simulink model "building_PHPP_v4"  (R2023b)
settings: Solver=ode23tb  StartTime=-building.preruntime+8760*3600  StopTime=building.runtime+8760*3600  EnableMultiTasking=on
PreLoadFcn:
  | tic
StartFcn:
  | pre_time = toc
  | assignin('base','pre_time',pre_time)
  | tic
StopFcn:
  | time = toc
  | assignin('base','time',time)
values from neighbouring files (symbols this model uses):
  A = 7*10*2    (= 140)    [theta_ground_v1.m]    (also in xlswrite1.m = num2cell(data))
  B = A/(0.5 * P)    (= 8.23529411765)    [theta_ground_v1.m]
  building = obj    [BUILDING.m]    (also in create_building_automatic.m = building.save(); ini_building_automatic.m = building.add_variant_hvac(building.variant_hvac, hvac); load_building_automatic.m = building.save())
  C = zeros(1,length(d)+1)    [CONSTRUCTION.m]    (also in DOOR.m = [0 0 0]; WALL.m = [0 0 0]; WINDOW.m = [0 0 0])
  cp = str2num(value)    [CONSTRUCTION.m]
  p = [timevec_weather weather(:,12)]    [BOUNDARY.m]    (also in WEATHER.m = 0; init_carnotUIBK.m = cell2mat(carnotUIBKpaths(i,2)))
  rho = str2num(value)    [CONSTRUCTION.m]    (also in theta_ground_v1.m = 2000)
undefined symbols (not defined in the file or in its folder): Dd, Dreifach, get_building, Qdot_C, Qdot_C_energy, Qdot_H, Qdot_H_energy, Qdot_I_electricity, Qdot_I_electricity_energy, Qdot_I_light, Qdot_I_light_energy, Qdot_I_person, Qdot_I_person_energy, Qdot_S, Qdot_S_energy, Qdot_T_ground, Qdot_T_ground_energy, Qdot_T_neighbour, Qdot_T_neighbour_energy, Qdot_T_opaque, Qdot_T_opaque_energy, Qdot_T_window, Qdot_T_window_energy, Qdot_V_infiltration, Qdot_V_infiltration_energy, Qdot_V_mech, Qdot_V_mech_energy, Qdot_V_window, Qdot_V_window_energy, Tc, Tr, Ts, Wärmeschutzglas, x_CO2, x_H2O, x_VOC
libraries: carnotUIBK x1874, carnot x9, simulink x6
(part 18 of 30)

== system building_PHPP_v4/BUILDING/INTERSECTION_8_9/wall_3 ==
  AIB1 : Inport
  AIB2 : Inport  Port=2
  Qdot_sol1 : Inport  Port=3
  Qdot_sol2 : Inport  Port=4
  EMPTY : carnotUIBK/wall_intersection/EMPTY  VariantControl=(default)
  R-C model : carnotUIBK/wall_intersection/R-C model  VariantControl=V_i_8_9_w3_m1  t0=z.t_ini  d=fliplr(const.parameter.xmesh_beu)  cond=fliplr(const.parameter.lambda)  cwall=fliplr(const.parameter.cp)  rho=fliplr(const.parameter.rho)  reflectground=0.2  abs_emiss=[const.absorption_2 const.emission_2 const.emission_1]  tau=const.parameter.tau  dactive=const.parameter.d_active
      link override alpha_i1/alpha_i_down: VariantControl=V_i_8_9_w3_hti2
      link override alpha_i1/alpha_i_horizontal: VariantControl=V_i_8_9_w3_hti0
      link override alpha_i1/alpha_i_up: VariantControl=V_i_8_9_w3_hti1
      link override alpha_i2/alpha_i_down: VariantControl=V_i_8_9_w3_hti2
      link override alpha_i2/alpha_i_horizontal: VariantControl=V_i_8_9_w3_hti0
      link override alpha_i2/alpha_i_up: VariantControl=V_i_8_9_w3_hti1
  UA : carnotUIBK/wall_intersection/UA  VariantControl=V_i_8_9_w3_m0  U=const.parameter.U
      link override Rsi/down: VariantControl=V_i_8_9_w3_hti2
      link override Rsi/horizontal: VariantControl=V_i_8_9_w3_hti0
      link override Rsi/up: VariantControl=V_i_8_9_w3_hti1
  hygrothermal model : carnotUIBK/wall_intersection/hygrothermal model  VariantControl=V_i_8_9_w3_m2  t0=z.t_ini  reflectground=0.2  abs_emiss=[const.absorption_2 const.emission_2 const.emission_1]  xmesh=const.parameter.xmesh_hygro  X=const.parameter.X  d=const.parameter.d  lambda=const.parameter.lambda_hygro  rho=const.parameter.rho_hygro  cp=const.parameter.cp_hygro  mu=const.parameter.mu  ufs=const.parameter.ufs  FSF_u=const.parameter.FSF_u  FSF_phi=const.parameter.FSF_phi  FSF_dudphi=const.parameter.FSF_dudphi  FSF_k=const.parameter.FSF_k  K_kleff=const.parameter.K_kleff  K_u=const.parameter.K_u  K_kl=const.parameter.K_kl  FSF_length=const.parameter.FSF_length  K_length=const.parameter.K_length  T_ini=const.parameter.T_ini_hygro  Phi_ini=const.parameter.Phi_ini_hygro  T_source=const.parameter.T_source  Phi_source=const.parameter.Phi_source  Tdactive=const.parameter.T_dactive  Phidactive=const.parameter.Phi_dactive
      link override alpha_i1/alpha_i_down: VariantControl=V_i_8_9_w3_hti2
      link override alpha_i1/alpha_i_horizontal: VariantControl=V_i_8_9_w3_hti0
      link override alpha_i1/alpha_i_up: VariantControl=V_i_8_9_w3_hti1
      link override alpha_i2/alpha_i_down: VariantControl=V_i_8_9_w3_hti2
      link override alpha_i2/alpha_i_horizontal: VariantControl=V_i_8_9_w3_hti0
      link override alpha_i2/alpha_i_up: VariantControl=V_i_8_9_w3_hti1
  "[S1]" : Outport  VectorParamsAs1DForOutWhenUnconnected=off
  "[S2]" : Outport  Port=2  VectorParamsAs1DForOutWhenUnconnected=off

== system building_PHPP_v4/BUILDING/INTERSECTION_9_10/airexchange_1 ==
  AIB1 : Inport
  AIB2 : Inport  Port=2
  control : Inport  Port=3
  EMPTY : carnotUIBK/airexchange_intersection/EMPTY  VariantControl=(default)
  airexchange_empiric : carnotUIBK/airexchange_intersection/airexchange_empiric  VariantControl=V_i_9_10_inf1_m0
  airexchange_powerlaw : carnotUIBK/airexchange_intersection/airexchange_powerlaw  VariantControl=V_i_9_10_inf1_m1
  "[S1]" : Outport  VectorParamsAs1DForOutWhenUnconnected=off
  "[S2]" : Outport  Port=2  VectorParamsAs1DForOutWhenUnconnected=off

== system building_PHPP_v4/BUILDING/INTERSECTION_9_10/airexchange_2 ==
  AIB1 : Inport
  AIB2 : Inport  Port=2
  control : Inport  Port=3
  EMPTY : carnotUIBK/airexchange_intersection/EMPTY  VariantControl=(default)
  airexchange_empiric : carnotUIBK/airexchange_intersection/airexchange_empiric  VariantControl=V_i_9_10_inf2_m0
  airexchange_powerlaw : carnotUIBK/airexchange_intersection/airexchange_powerlaw  VariantControl=V_i_9_10_inf2_m1
  "[S1]" : Outport  VectorParamsAs1DForOutWhenUnconnected=off
  "[S2]" : Outport  Port=2  VectorParamsAs1DForOutWhenUnconnected=off

== system building_PHPP_v4/BUILDING/INTERSECTION_9_10/airexchange_3 ==
  AIB1 : Inport
  AIB2 : Inport  Port=2
  control : Inport  Port=3
  EMPTY : carnotUIBK/airexchange_intersection/EMPTY  VariantControl=(default)
  airexchange_empiric : carnotUIBK/airexchange_intersection/airexchange_empiric  VariantControl=V_i_9_10_inf3_m0
  airexchange_powerlaw : carnotUIBK/airexchange_intersection/airexchange_powerlaw  VariantControl=V_i_9_10_inf3_m1
  "[S1]" : Outport  VectorParamsAs1DForOutWhenUnconnected=off
  "[S2]" : Outport  Port=2  VectorParamsAs1DForOutWhenUnconnected=off

== system building_PHPP_v4/BUILDING/INTERSECTION_9_10/wall_1 ==
  AIB1 : Inport
  AIB2 : Inport  Port=2
  Qdot_sol1 : Inport  Port=3
  Qdot_sol2 : Inport  Port=4
  EMPTY : carnotUIBK/wall_intersection/EMPTY  VariantControl=(default)
  R-C model : carnotUIBK/wall_intersection/R-C model  VariantControl=V_i_9_10_w1_m1  t0=z.t_ini  d=fliplr(const.parameter.xmesh_beu)  cond=fliplr(const.parameter.lambda)  cwall=fliplr(const.parameter.cp)  rho=fliplr(const.parameter.rho)  reflectground=0.2  abs_emiss=[const.absorption_2 const.emission_2 const.emission_1]  tau=const.parameter.tau  dactive=const.parameter.d_active
      link override alpha_i1/alpha_i_down: VariantControl=V_i_9_10_w1_hti2
      link override alpha_i1/alpha_i_horizontal: VariantControl=V_i_9_10_w1_hti0
      link override alpha_i1/alpha_i_up: VariantControl=V_i_9_10_w1_hti1
      link override alpha_i2/alpha_i_down: VariantControl=V_i_9_10_w1_hti2
      link override alpha_i2/alpha_i_horizontal: VariantControl=V_i_9_10_w1_hti0
      link override alpha_i2/alpha_i_up: VariantControl=V_i_9_10_w1_hti1
  UA : carnotUIBK/wall_intersection/UA  VariantControl=V_i_9_10_w1_m0  U=const.parameter.U
      link override Rsi/down: VariantControl=V_i_9_10_w1_hti2
      link override Rsi/horizontal: VariantControl=V_i_9_10_w1_hti0
      link override Rsi/up: VariantControl=V_i_9_10_w1_hti1
  hygrothermal model : carnotUIBK/wall_intersection/hygrothermal model  VariantControl=V_i_9_10_w1_m2  t0=z.t_ini  reflectground=0.2  abs_emiss=[const.absorption_2 const.emission_2 const.emission_1]  xmesh=const.parameter.xmesh_hygro  X=const.parameter.X  d=const.parameter.d  lambda=const.parameter.lambda_hygro  rho=const.parameter.rho_hygro  cp=const.parameter.cp_hygro  mu=const.parameter.mu  ufs=const.parameter.ufs  FSF_u=const.parameter.FSF_u  FSF_phi=const.parameter.FSF_phi  FSF_dudphi=const.parameter.FSF_dudphi  FSF_k=const.parameter.FSF_k  K_kleff=const.parameter.K_kleff  K_u=const.parameter.K_u  K_kl=const.parameter.K_kl  FSF_length=const.parameter.FSF_length  K_length=const.parameter.K_length  T_ini=const.parameter.T_ini_hygro  Phi_ini=const.parameter.Phi_ini_hygro  T_source=const.parameter.T_source  Phi_source=const.parameter.Phi_source  Tdactive=const.parameter.T_dactive  Phidactive=const.parameter.Phi_dactive
      link override alpha_i1/alpha_i_down: VariantControl=V_i_9_10_w1_hti2
      link override alpha_i1/alpha_i_horizontal: VariantControl=V_i_9_10_w1_hti0
      link override alpha_i1/alpha_i_up: VariantControl=V_i_9_10_w1_hti1
      link override alpha_i2/alpha_i_down: VariantControl=V_i_9_10_w1_hti2
      link override alpha_i2/alpha_i_horizontal: VariantControl=V_i_9_10_w1_hti0
      link override alpha_i2/alpha_i_up: VariantControl=V_i_9_10_w1_hti1
  "[S1]" : Outport  VectorParamsAs1DForOutWhenUnconnected=off
  "[S2]" : Outport  Port=2  VectorParamsAs1DForOutWhenUnconnected=off

== system building_PHPP_v4/BUILDING/INTERSECTION_9_10/wall_2 ==
  AIB1 : Inport
  AIB2 : Inport  Port=2
  Qdot_sol1 : Inport  Port=3
  Qdot_sol2 : Inport  Port=4
  EMPTY : carnotUIBK/wall_intersection/EMPTY  VariantControl=(default)
  R-C model : carnotUIBK/wall_intersection/R-C model  VariantControl=V_i_9_10_w2_m1  t0=z.t_ini  d=fliplr(const.parameter.xmesh_beu)  cond=fliplr(const.parameter.lambda)  cwall=fliplr(const.parameter.cp)  rho=fliplr(const.parameter.rho)  reflectground=0.2  abs_emiss=[const.absorption_2 const.emission_2 const.emission_1]  tau=const.parameter.tau  dactive=const.parameter.d_active
      link override alpha_i1/alpha_i_down: VariantControl=V_i_9_10_w2_hti2
      link override alpha_i1/alpha_i_horizontal: VariantControl=V_i_9_10_w2_hti0
      link override alpha_i1/alpha_i_up: VariantControl=V_i_9_10_w2_hti1
      link override alpha_i2/alpha_i_down: VariantControl=V_i_9_10_w2_hti2
      link override alpha_i2/alpha_i_horizontal: VariantControl=V_i_9_10_w2_hti0
      link override alpha_i2/alpha_i_up: VariantControl=V_i_9_10_w2_hti1
  UA : carnotUIBK/wall_intersection/UA  VariantControl=V_i_9_10_w2_m0  U=const.parameter.U
      link override Rsi/down: VariantControl=V_i_9_10_w2_hti2
      link override Rsi/horizontal: VariantControl=V_i_9_10_w2_hti0
      link override Rsi/up: VariantControl=V_i_9_10_w2_hti1
  hygrothermal model : carnotUIBK/wall_intersection/hygrothermal model  VariantControl=V_i_9_10_w2_m2  t0=z.t_ini  reflectground=0.2  abs_emiss=[const.absorption_2 const.emission_2 const.emission_1]  xmesh=const.parameter.xmesh_hygro  X=const.parameter.X  d=const.parameter.d  lambda=const.parameter.lambda_hygro  rho=const.parameter.rho_hygro  cp=const.parameter.cp_hygro  mu=const.parameter.mu  ufs=const.parameter.ufs  FSF_u=const.parameter.FSF_u  FSF_phi=const.parameter.FSF_phi  FSF_dudphi=const.parameter.FSF_dudphi  FSF_k=const.parameter.FSF_k  K_kleff=const.parameter.K_kleff  K_u=const.parameter.K_u  K_kl=const.parameter.K_kl  FSF_length=const.parameter.FSF_length  K_length=const.parameter.K_length  T_ini=const.parameter.T_ini_hygro  Phi_ini=const.parameter.Phi_ini_hygro  T_source=const.parameter.T_source  Phi_source=const.parameter.Phi_source  Tdactive=const.parameter.T_dactive  Phidactive=const.parameter.Phi_dactive
      link override alpha_i1/alpha_i_down: VariantControl=V_i_9_10_w2_hti2
      link override alpha_i1/alpha_i_horizontal: VariantControl=V_i_9_10_w2_hti0
      link override alpha_i1/alpha_i_up: VariantControl=V_i_9_10_w2_hti1
      link override alpha_i2/alpha_i_down: VariantControl=V_i_9_10_w2_hti2
      link override alpha_i2/alpha_i_horizontal: VariantControl=V_i_9_10_w2_hti0
      link override alpha_i2/alpha_i_up: VariantControl=V_i_9_10_w2_hti1
  "[S1]" : Outport  VectorParamsAs1DForOutWhenUnconnected=off
  "[S2]" : Outport  Port=2  VectorParamsAs1DForOutWhenUnconnected=off

== system building_PHPP_v4/BUILDING/INTERSECTION_9_10/wall_3 ==
  AIB1 : Inport
  AIB2 : Inport  Port=2
  Qdot_sol1 : Inport  Port=3
  Qdot_sol2 : Inport  Port=4
  EMPTY : carnotUIBK/wall_intersection/EMPTY  VariantControl=(default)
  R-C model : carnotUIBK/wall_intersection/R-C model  VariantControl=V_i_9_10_w3_m1  t0=z.t_ini  d=fliplr(const.parameter.xmesh_beu)  cond=fliplr(const.parameter.lambda)  cwall=fliplr(const.parameter.cp)  rho=fliplr(const.parameter.rho)  reflectground=0.2  abs_emiss=[const.absorption_2 const.emission_2 const.emission_1]  tau=const.parameter.tau  dactive=const.parameter.d_active
      link override alpha_i1/alpha_i_down: VariantControl=V_i_9_10_w3_hti2
      link override alpha_i1/alpha_i_horizontal: VariantControl=V_i_9_10_w3_hti0
      link override alpha_i1/alpha_i_up: VariantControl=V_i_9_10_w3_hti1
      link override alpha_i2/alpha_i_down: VariantControl=V_i_9_10_w3_hti2
      link override alpha_i2/alpha_i_horizontal: VariantControl=V_i_9_10_w3_hti0
      link override alpha_i2/alpha_i_up: VariantControl=V_i_9_10_w3_hti1
  UA : carnotUIBK/wall_intersection/UA  VariantControl=V_i_9_10_w3_m0  U=const.parameter.U
      link override Rsi/down: VariantControl=V_i_9_10_w3_hti2
      link override Rsi/horizontal: VariantControl=V_i_9_10_w3_hti0
      link override Rsi/up: VariantControl=V_i_9_10_w3_hti1
  hygrothermal model : carnotUIBK/wall_intersection/hygrothermal model  VariantControl=V_i_9_10_w3_m2  t0=z.t_ini  reflectground=0.2  abs_emiss=[const.absorption_2 const.emission_2 const.emission_1]  xmesh=const.parameter.xmesh_hygro  X=const.parameter.X  d=const.parameter.d  lambda=const.parameter.lambda_hygro  rho=const.parameter.rho_hygro  cp=const.parameter.cp_hygro  mu=const.parameter.mu  ufs=const.parameter.ufs  FSF_u=const.parameter.FSF_u  FSF_phi=const.parameter.FSF_phi  FSF_dudphi=const.parameter.FSF_dudphi  FSF_k=const.parameter.FSF_k  K_kleff=const.parameter.K_kleff  K_u=const.parameter.K_u  K_kl=const.parameter.K_kl  FSF_length=const.parameter.FSF_length  K_length=const.parameter.K_length  T_ini=const.parameter.T_ini_hygro  Phi_ini=const.parameter.Phi_ini_hygro  T_source=const.parameter.T_source  Phi_source=const.parameter.Phi_source  Tdactive=const.parameter.T_dactive  Phidactive=const.parameter.Phi_dactive
      link override alpha_i1/alpha_i_down: VariantControl=V_i_9_10_w3_hti2
      link override alpha_i1/alpha_i_horizontal: VariantControl=V_i_9_10_w3_hti0
      link override alpha_i1/alpha_i_up: VariantControl=V_i_9_10_w3_hti1
      link override alpha_i2/alpha_i_down: VariantControl=V_i_9_10_w3_hti2
      link override alpha_i2/alpha_i_horizontal: VariantControl=V_i_9_10_w3_hti0
      link override alpha_i2/alpha_i_up: VariantControl=V_i_9_10_w3_hti1
  "[S1]" : Outport  VectorParamsAs1DForOutWhenUnconnected=off
  "[S2]" : Outport  Port=2  VectorParamsAs1DForOutWhenUnconnected=off

== system building_PHPP_v4/BUILDING/ZONE_1/gain_1 ==
  AIB : Inport
  control : Inport  Port=2
  EMPTY : carnotUIBK/gain/EMPTY  SystemSampleTime=-1  VariantControl=(default)
  Equipment : carnotUIBK/gain/Equipment  SystemSampleTime=-1  VariantControl=V_z1_i1_m2
  Light : carnotUIBK/gain/Light  SystemSampleTime=-1  VariantControl=V_z1_i1_m1
  Moisture : carnotUIBK/gain/Moisture  SystemSampleTime=-1  VariantControl=V_z1_i1_m3
  People : carnotUIBK/gain/People  SystemSampleTime=-1  VariantControl=V_z1_i1_m0  VariantActivationTime=update diagram  AllowFlexibleInterface=on  Latency=0  AutoFrameSizeCalculation=off
  "[S]" : Outport  VectorParamsAs1DForOutWhenUnconnected=off

== system building_PHPP_v4/BUILDING/ZONE_1/gain_2 ==
  AIB : Inport
  control : Inport  Port=2
  EMPTY : carnotUIBK/gain/EMPTY  SystemSampleTime=-1  VariantControl=(default)  VariantActivationTime=update diagram  AllowFlexibleInterface=on  Latency=0  AutoFrameSizeCalculation=off
  Equipment : carnotUIBK/gain/Equipment  SystemSampleTime=-1  VariantControl=V_z1_i2_m2
  Light : carnotUIBK/gain/Light  SystemSampleTime=-1  VariantControl=V_z1_i2_m1
  Moisture : carnotUIBK/gain/Moisture  SystemSampleTime=-1  VariantControl=V_z1_i2_m3
  People : carnotUIBK/gain/People  SystemSampleTime=-1  VariantControl=V_z1_i2_m0
  "[S]" : Outport  VectorParamsAs1DForOutWhenUnconnected=off

== system building_PHPP_v4/BUILDING/ZONE_1/gain_3 ==
  AIB : Inport
  control : Inport  Port=2
  EMPTY : carnotUIBK/gain/EMPTY  SystemSampleTime=-1  VariantControl=(default)  VariantActivationTime=update diagram  AllowFlexibleInterface=on  Latency=0  AutoFrameSizeCalculation=off
  Equipment : carnotUIBK/gain/Equipment  SystemSampleTime=-1  VariantControl=V_z1_i3_m2
  Light : carnotUIBK/gain/Light  SystemSampleTime=-1  VariantControl=V_z1_i3_m1
  Moisture : carnotUIBK/gain/Moisture  SystemSampleTime=-1  VariantControl=V_z1_i3_m3
  People : carnotUIBK/gain/People  SystemSampleTime=-1  VariantControl=V_z1_i3_m0
  "[S]" : Outport  VectorParamsAs1DForOutWhenUnconnected=off

== system building_PHPP_v4/BUILDING/ZONE_1/gain_4 ==
  AIB : Inport
  control : Inport  Port=2
  EMPTY : carnotUIBK/gain/EMPTY  SystemSampleTime=-1  VariantControl=(default)  VariantActivationTime=update diagram  AllowFlexibleInterface=on  Latency=0  AutoFrameSizeCalculation=off
  Equipment : carnotUIBK/gain/Equipment  SystemSampleTime=-1  VariantControl=V_z1_i4_m2
  Light : carnotUIBK/gain/Light  SystemSampleTime=-1  VariantControl=V_z1_i4_m1
  Moisture : carnotUIBK/gain/Moisture  SystemSampleTime=-1  VariantControl=V_z1_i4_m3
  People : carnotUIBK/gain/People  SystemSampleTime=-1  VariantControl=V_z1_i4_m0
  "[S]" : Outport  VectorParamsAs1DForOutWhenUnconnected=off

== system building_PHPP_v4/BUILDING/ZONE_1/gain_5 ==
  AIB : Inport
  control : Inport  Port=2
  EMPTY : carnotUIBK/gain/EMPTY  SystemSampleTime=-1  VariantControl=(default)  VariantActivationTime=update diagram  AllowFlexibleInterface=on  Latency=0  AutoFrameSizeCalculation=off
  Equipment : carnotUIBK/gain/Equipment  SystemSampleTime=-1  VariantControl=V_z1_i5_m2
  Light : carnotUIBK/gain/Light  SystemSampleTime=-1  VariantControl=V_z1_i5_m1
  Moisture : carnotUIBK/gain/Moisture  SystemSampleTime=-1  VariantControl=V_z1_i5_m3
  People : carnotUIBK/gain/People  SystemSampleTime=-1  VariantControl=V_z1_i5_m0
  "[S]" : Outport  VectorParamsAs1DForOutWhenUnconnected=off

== system building_PHPP_v4/BUILDING/ZONE_1/infiltration_1 ==
  AIB : Inport
  WDB : Inport  Port=2
  control : Inport  Port=3
  EMPTY : carnotUIBK/infiltration/EMPTY  VariantControl=(default)
  infiltration_constant : carnotUIBK/infiltration/infiltration_constant  VariantControl=V_z1_inf1_m0  volume=z.heated_volume  n50=z.n50  wind_e=0.07  co2=400
  infiltration_pressure : carnotUIBK/infiltration/infiltration_pressure  VariantControl=V_z1_inf1_m1  volume=z.heated_volume  n50=z.n50  wind_e=0.07  co2=400
  "[S]" : Outport  VectorParamsAs1DForOutWhenUnconnected=off

== system building_PHPP_v4/BUILDING/ZONE_1/infiltration_2 ==
  AIB : Inport
  WDB : Inport  Port=2
  control : Inport  Port=3
  EMPTY : carnotUIBK/infiltration/EMPTY  VariantControl=(default)
  infiltration_constant : carnotUIBK/infiltration/infiltration_constant  VariantControl=V_z1_inf2_m0  volume=z.heated_volume  n50=z.n50  wind_e=0.07  co2=400
  infiltration_pressure : carnotUIBK/infiltration/infiltration_pressure  VariantControl=V_z1_inf2_m1  volume=z.heated_volume  n50=z.n50  wind_e=0.07  co2=400
  "[S]" : Outport  VectorParamsAs1DForOutWhenUnconnected=off

== system building_PHPP_v4/BUILDING/ZONE_1/infiltration_3 ==
  AIB : Inport
  WDB : Inport  Port=2
  control : Inport  Port=3
  EMPTY : carnotUIBK/infiltration/EMPTY  VariantControl=(default)
  infiltration_constant : carnotUIBK/infiltration/infiltration_constant  VariantControl=V_z1_inf3_m0  volume=z.heated_volume  n50=z.n50  wind_e=0.07  co2=400
  infiltration_pressure : carnotUIBK/infiltration/infiltration_pressure  VariantControl=V_z1_inf3_m1  volume=z.heated_volume  n50=z.n50  wind_e=0.07  co2=400
  "[S]" : Outport  VectorParamsAs1DForOutWhenUnconnected=off

== system building_PHPP_v4/BUILDING/ZONE_1/infiltration_4 ==
  AIB : Inport
  WDB : Inport  Port=2
  control : Inport  Port=3
  EMPTY : carnotUIBK/infiltration/EMPTY  VariantControl=(default)
  infiltration_constant : carnotUIBK/infiltration/infiltration_constant  VariantControl=V_z1_inf4_m0  volume=z.heated_volume  n50=z.n50  wind_e=0.07  co2=400
  infiltration_pressure : carnotUIBK/infiltration/infiltration_pressure  VariantControl=V_z1_inf4_m1  volume=z.heated_volume  n50=z.n50  wind_e=0.07  co2=400
  "[S]" : Outport  VectorParamsAs1DForOutWhenUnconnected=off

== system building_PHPP_v4/BUILDING/ZONE_1/infiltration_5 ==
  AIB : Inport
  WDB : Inport  Port=2
  control : Inport  Port=3
  EMPTY : carnotUIBK/infiltration/EMPTY  VariantControl=(default)
  infiltration_constant : carnotUIBK/infiltration/infiltration_constant  VariantControl=V_z1_inf5_m0  volume=z.heated_volume  n50=z.n50  wind_e=0.07  co2=400
  infiltration_pressure : carnotUIBK/infiltration/infiltration_pressure  VariantControl=V_z1_inf5_m1  volume=z.heated_volume  n50=z.n50  wind_e=0.07  co2=400
  "[S]" : Outport  VectorParamsAs1DForOutWhenUnconnected=off

== system building_PHPP_v4/BUILDING/ZONE_1/room_node ==
  sum([S]) : Inport
  1-node : carnotUIBK/room_node/1-node  VariantControl=V_z1_m2  zoneairvolume=z.heated_volume  zoneheight=z.heated_volume/z.heated_area  zonestartTEMP=z.t_ini  zonestartWATER=z.phi_ini  zonestartCO2=z.CO2_ini  zonestartVOC=z.VOC_ini  zonestartP0=1e5/(293.15)*(273.15+z.t_ini)  timeconst=z.timeconstant  mcp=z.cp_spec*z.heated_area
  1-node_womass : carnotUIBK/room_node/1-node_womass  VariantControl=V_z1_m4  zoneairvolume=z.heated_volume  zoneheight=z.heated_volume/z.heated_area  zonestartTEMP=z.t_ini  zonestartWATER=z.phi_ini  zonestartCO2=z.CO2_ini  zonestartVOC=z.VOC_ini  zonestartP0=1e5/(293.15)*(273.15+z.t_ini)  timeconst=z.timeconstant  mcp=z.cp_spec*z.heated_area
  2-node : carnotUIBK/room_node/2-node  VariantControl=V_z1_m3  zoneairvolume=z.heated_volume  zoneheight=z.heated_volume/z.heated_area  zonestartTEMP=z.t_ini  zonestartWATER=z.phi_ini  zonestartCO2=z.CO2_ini  zonestartVOC=z.VOC_ini  zonestartP0=1e5/(293.15)*(273.15+z.t_ini)  timeconst=z.timeconstant
  2-node_ideal : carnotUIBK/room_node/2-node_ideal  VariantControl=V_z1_m1  zoneairvolume=z.heated_volume  zoneheight=z.heated_volume/z.heated_area  zonestartTEMP=z.t_ini  zonestartWATER=z.phi_ini  zonestartCO2=z.CO2_ini  zonestartVOC=z.VOC_ini  zonestartP0=1e5/(293.15)*(273.15+z.t_ini)  timeconst=z.timeconstant  temperature_timevalues=z.profile_timevalues  temperature_timeduration=z.profile_timeduration  temperature_Tc=z.profile_Tc  temperature_Tr=z.profile_Tc
  EMPTY : carnotUIBK/room_node/EMPTY  VariantControl=(default)  temperature_timevalues=z.profile_timevalues  temperature_timeduration=z.profile_timeduration  temperature_Tc=z.profile_Tc  temperature_Tr=z.profile_Tr  temperature_rH=z.profile_rH  temperature_CO2=z.profile_CO2  temperature_VOC=z.profile_VOC  temperature_p=z.profile_p
  BDB : Outport  VectorParamsAs1DForOutWhenUnconnected=off
  AIB : Outport  Port=2  VectorParamsAs1DForOutWhenUnconnected=off
  Qdot_sol : Outport  Port=3  VectorParamsAs1DForOutWhenUnconnected=off

== system building_PHPP_v4/BUILDING/ZONE_1/wall_1 ==
  WDB : Inport
  GDB : Inport  Port=2
  NDB : Inport  Port=3
  AIB : Inport  Port=4
  Qdot_in : Inport  Port=5
  Qdot_sol : Inport  Port=6
  EMPTY : carnotUIBK/wall_zone/EMPTY  VariantControl=(default)
  R-C model : carnotUIBK/wall_zone/R-C model  VariantControl=V_z1_w1_m1  t0=z.t_ini  d=fliplr(const.parameter.xmesh_beu)  cond=fliplr(const.parameter.lambda)  cwall=fliplr(const.parameter.cp)  rho=fliplr(const.parameter.rho)  reflectground=0.2  abs_emiss=[const.absorption_2 const.emission_2 const.emission_1]  tau=const.parameter.tau  dactive=const.parameter.d_active
      link override alpha_e/alpha_e_AMBIENT: VariantControl=V_z1_w1_hte0
      link override alpha_e/alpha_e_GROUND: VariantControl=V_z1_w1_hte1
      link override alpha_e/alpha_e_INTERNAL: VariantControl=V_z1_w1_hte2
      link override alpha_e/alpha_e_INTERNAL/alpha_i/alpha_i_down: VariantControl=V_z1_w1_hti2
      link override alpha_e/alpha_e_INTERNAL/alpha_i/alpha_i_horizontal: VariantControl=V_z1_w1_hti0
      link override alpha_e/alpha_e_INTERNAL/alpha_i/alpha_i_up: VariantControl=V_z1_w1_hti1
      link override alpha_e/alpha_e_NEIGHBOUR: VariantControl=V_z1_w1_hte3
      link override alpha_e/alpha_e_NEIGHBOUR/alpha_i/alpha_i_down: VariantControl=V_z1_w1_hti2
      link override alpha_e/alpha_e_NEIGHBOUR/alpha_i/alpha_i_horizontal: VariantControl=V_z1_w1_hti0
      link override alpha_e/alpha_e_NEIGHBOUR/alpha_i/alpha_i_up: VariantControl=V_z1_w1_hti1
      link override alpha_i/alpha_i_down: VariantControl=V_z1_w1_hti2
      link override alpha_i/alpha_i_horizontal: VariantControl=V_z1_w1_hti0
      link override alpha_i/alpha_i_up: VariantControl=V_z1_w1_hti1
  UA : carnotUIBK/wall_zone/UA  VariantControl=V_z1_w1_m0  U=const.parameter.U
      link override Rse/AMBIENT: VariantControl=V_z1_w1_hte0
      link override Rse/GROUND: VariantControl=V_z1_w1_hte1
      link override Rse/INTERNAL: VariantControl=V_z1_w1_hte2
      link override Rse/NEIGHBOUR: VariantControl=V_z1_w1_hte3
      link override Rsi/down: VariantControl=V_z1_w1_hti2
      link override Rsi/horizontal: VariantControl=V_z1_w1_hti0
      link override Rsi/up: VariantControl=V_z1_w1_hti1
  hygrothermal model : carnotUIBK/wall_zone/hygrothermal model  VariantControl=V_z1_w1_m2  t0=z.t_ini  reflectground=0.2  abs_emiss=[const.absorption_2 const.emission_2 const.emission_1]  xmesh=const.parameter.xmesh_hygro  X=const.parameter.X  d=const.parameter.d  lambda=const.parameter.lambda_hygro  rho=const.parameter.rho_hygro  cp=const.parameter.cp_hygro  mu=const.parameter.mu  ufs=const.parameter.ufs  FSF_u=const.parameter.FSF_u  FSF_phi=const.parameter.FSF_phi  FSF_dudphi=const.parameter.FSF_dudphi  FSF_k=const.parameter.FSF_k  K_kleff=const.parameter.K_kleff  K_u=const.parameter.K_u  K_kl=const.parameter.K_kl  FSF_length=const.parameter.FSF_length  K_length=const.parameter.K_length  T_ini=const.parameter.T_ini_hygro  Phi_ini=const.parameter.Phi_ini_hygro  T_source=const.parameter.T_source  Phi_source=const.parameter.Phi_source  Tdactive=const.parameter.T_dactive  Phidactive=const.parameter.Phi_dactive
      link override alpha_e/alpha_e_AMBIENT: VariantControl=V_z1_w1_hte0
      link override alpha_e/alpha_e_GROUND: VariantControl=V_z1_w1_hte1
      link override alpha_e/alpha_e_INTERNAL: VariantControl=V_z1_w1_hte2
      link override alpha_e/alpha_e_INTERNAL/alpha_i/alpha_i_down: VariantControl=V_z1_w1_hti2
      link override alpha_e/alpha_e_INTERNAL/alpha_i/alpha_i_horizontal: VariantControl=V_z1_w1_hti0
      link override alpha_e/alpha_e_INTERNAL/alpha_i/alpha_i_up: VariantControl=V_z1_w1_hti1
      link override alpha_e/alpha_e_NEIGHBOUR: VariantControl=V_z1_w1_hte3
      link override alpha_e/alpha_e_NEIGHBOUR/alpha_i/alpha_i_down: VariantControl=V_z1_w1_hti2
      link override alpha_e/alpha_e_NEIGHBOUR/alpha_i/alpha_i_horizontal: VariantControl=V_z1_w1_hti0
      link override alpha_e/alpha_e_NEIGHBOUR/alpha_i/alpha_i_up: VariantControl=V_z1_w1_hti1
      link override alpha_i/alpha_i_down: VariantControl=V_z1_w1_hti2
      link override alpha_i/alpha_i_horizontal: VariantControl=V_z1_w1_hti0
      link override alpha_i/alpha_i_up: VariantControl=V_z1_w1_hti1
  "[S]" : Outport  VectorParamsAs1DForOutWhenUnconnected=off
  theta_out : Outport  Port=2  VectorParamsAs1DForOutWhenUnconnected=off

== system building_PHPP_v4/BUILDING/ZONE_1/wall_10 ==
  WDB : Inport
  GDB : Inport  Port=2
  NDB : Inport  Port=3
  AIB : Inport  Port=4
  Qdot_in : Inport  Port=5
  Qdot_sol : Inport  Port=6
  EMPTY : carnotUIBK/wall_zone/EMPTY  VariantControl=(default)
  R-C model : carnotUIBK/wall_zone/R-C model  VariantControl=V_z1_w10_m1  t0=z.t_ini  d=fliplr(const.parameter.xmesh_beu)  cond=fliplr(const.parameter.lambda)  cwall=fliplr(const.parameter.cp)  rho=fliplr(const.parameter.rho)  reflectground=0.2  abs_emiss=[const.absorption_2 const.emission_2 const.emission_1]  tau=const.parameter.tau  dactive=const.parameter.d_active
      link override alpha_e/alpha_e_AMBIENT: VariantControl=V_z1_w10_hte0
      link override alpha_e/alpha_e_GROUND: VariantControl=V_z1_w10_hte1
      link override alpha_e/alpha_e_INTERNAL: VariantControl=V_z1_w10_hte2
      link override alpha_e/alpha_e_INTERNAL/alpha_i/alpha_i_down: VariantControl=V_z1_w10_hti2
      link override alpha_e/alpha_e_INTERNAL/alpha_i/alpha_i_horizontal: VariantControl=V_z1_w10_hti0
      link override alpha_e/alpha_e_INTERNAL/alpha_i/alpha_i_up: VariantControl=V_z1_w10_hti1
      link override alpha_e/alpha_e_NEIGHBOUR: VariantControl=V_z1_w10_hte3
      link override alpha_e/alpha_e_NEIGHBOUR/alpha_i/alpha_i_down: VariantControl=V_z1_w10_hti2
      link override alpha_e/alpha_e_NEIGHBOUR/alpha_i/alpha_i_horizontal: VariantControl=V_z1_w10_hti0
      link override alpha_e/alpha_e_NEIGHBOUR/alpha_i/alpha_i_up: VariantControl=V_z1_w10_hti1
      link override alpha_i/alpha_i_down: VariantControl=V_z1_w10_hti2
      link override alpha_i/alpha_i_horizontal: VariantControl=V_z1_w10_hti0
      link override alpha_i/alpha_i_up: VariantControl=V_z1_w10_hti1
  UA : carnotUIBK/wall_zone/UA  VariantControl=V_z1_w10_m0  U=const.parameter.U
      link override Rse/AMBIENT: VariantControl=V_z1_w10_hte0
      link override Rse/GROUND: VariantControl=V_z1_w10_hte1
      link override Rse/INTERNAL: VariantControl=V_z1_w10_hte2
      link override Rse/NEIGHBOUR: VariantControl=V_z1_w10_hte3
      link override Rsi/down: VariantControl=V_z1_w10_hti2
      link override Rsi/horizontal: VariantControl=V_z1_w10_hti0
      link override Rsi/up: VariantControl=V_z1_w10_hti1
  hygrothermal model : carnotUIBK/wall_zone/hygrothermal model  VariantControl=V_z1_w10_m2  t0=z.t_ini  reflectground=0.2  abs_emiss=[const.absorption_2 const.emission_2 const.emission_1]  xmesh=const.parameter.xmesh_hygro  X=const.parameter.X  d=const.parameter.d  lambda=const.parameter.lambda_hygro  rho=const.parameter.rho_hygro  cp=const.parameter.cp_hygro  mu=const.parameter.mu  ufs=const.parameter.ufs  FSF_u=const.parameter.FSF_u  FSF_phi=const.parameter.FSF_phi  FSF_dudphi=const.parameter.FSF_dudphi  FSF_k=const.parameter.FSF_k  K_kleff=const.parameter.K_kleff  K_u=const.parameter.K_u  K_kl=const.parameter.K_kl  FSF_length=const.parameter.FSF_length  K_length=const.parameter.K_length  T_ini=const.parameter.T_ini_hygro  Phi_ini=const.parameter.Phi_ini_hygro  T_source=const.parameter.T_source  Phi_source=const.parameter.Phi_source  Tdactive=const.parameter.T_dactive  Phidactive=const.parameter.Phi_dactive
      link override alpha_e/alpha_e_AMBIENT: VariantControl=V_z1_w10_hte0
      link override alpha_e/alpha_e_GROUND: VariantControl=V_z1_w10_hte1
      link override alpha_e/alpha_e_INTERNAL: VariantControl=V_z1_w10_hte2
      link override alpha_e/alpha_e_INTERNAL/alpha_i/alpha_i_down: VariantControl=V_z1_w10_hti2
      link override alpha_e/alpha_e_INTERNAL/alpha_i/alpha_i_horizontal: VariantControl=V_z1_w10_hti0
      link override alpha_e/alpha_e_INTERNAL/alpha_i/alpha_i_up: VariantControl=V_z1_w10_hti1
      link override alpha_e/alpha_e_NEIGHBOUR: VariantControl=V_z1_w10_hte3
      link override alpha_e/alpha_e_NEIGHBOUR/alpha_i/alpha_i_down: VariantControl=V_z1_w10_hti2
      link override alpha_e/alpha_e_NEIGHBOUR/alpha_i/alpha_i_horizontal: VariantControl=V_z1_w10_hti0
      link override alpha_e/alpha_e_NEIGHBOUR/alpha_i/alpha_i_up: VariantControl=V_z1_w10_hti1
      link override alpha_i/alpha_i_down: VariantControl=V_z1_w10_hti2
      link override alpha_i/alpha_i_horizontal: VariantControl=V_z1_w10_hti0
      link override alpha_i/alpha_i_up: VariantControl=V_z1_w10_hti1
  "[S]" : Outport  VectorParamsAs1DForOutWhenUnconnected=off
  theta_out : Outport  Port=2  VectorParamsAs1DForOutWhenUnconnected=off

== system building_PHPP_v4/BUILDING/ZONE_1/wall_2 ==
  WDB : Inport
  GDB : Inport  Port=2
  NDB : Inport  Port=3
  AIB : Inport  Port=4
  Qdot_in : Inport  Port=5
  Qdot_sol : Inport  Port=6
  EMPTY : carnotUIBK/wall_zone/EMPTY  VariantControl=(default)
  R-C model : carnotUIBK/wall_zone/R-C model  VariantControl=V_z1_w2_m1  t0=z.t_ini  d=fliplr(const.parameter.xmesh_beu)  cond=fliplr(const.parameter.lambda)  cwall=fliplr(const.parameter.cp)  rho=fliplr(const.parameter.rho)  reflectground=0.2  abs_emiss=[const.absorption_2 const.emission_2 const.emission_1]  tau=const.parameter.tau  dactive=const.parameter.d_active
      link override alpha_e/alpha_e_AMBIENT: VariantControl=V_z1_w2_hte0
      link override alpha_e/alpha_e_GROUND: VariantControl=V_z1_w2_hte1
      link override alpha_e/alpha_e_INTERNAL: VariantControl=V_z1_w2_hte2
      link override alpha_e/alpha_e_INTERNAL/alpha_i/alpha_i_down: VariantControl=V_z1_w2_hti2
      link override alpha_e/alpha_e_INTERNAL/alpha_i/alpha_i_horizontal: VariantControl=V_z1_w2_hti0
      link override alpha_e/alpha_e_INTERNAL/alpha_i/alpha_i_up: VariantControl=V_z1_w2_hti1
      link override alpha_e/alpha_e_NEIGHBOUR: VariantControl=V_z1_w2_hte3
      link override alpha_e/alpha_e_NEIGHBOUR/alpha_i/alpha_i_down: VariantControl=V_z1_w2_hti2
      link override alpha_e/alpha_e_NEIGHBOUR/alpha_i/alpha_i_horizontal: VariantControl=V_z1_w2_hti0
      link override alpha_e/alpha_e_NEIGHBOUR/alpha_i/alpha_i_up: VariantControl=V_z1_w2_hti1
      link override alpha_i/alpha_i_down: VariantControl=V_z1_w2_hti2
      link override alpha_i/alpha_i_horizontal: VariantControl=V_z1_w2_hti0
      link override alpha_i/alpha_i_up: VariantControl=V_z1_w2_hti1
  UA : carnotUIBK/wall_zone/UA  VariantControl=V_z1_w2_m0  U=const.parameter.U
      link override Rse/AMBIENT: VariantControl=V_z1_w2_hte0
      link override Rse/GROUND: VariantControl=V_z1_w2_hte1
      link override Rse/INTERNAL: VariantControl=V_z1_w2_hte2
      link override Rse/NEIGHBOUR: VariantControl=V_z1_w2_hte3
      link override Rsi/down: VariantControl=V_z1_w2_hti2
      link override Rsi/horizontal: VariantControl=V_z1_w2_hti0
      link override Rsi/up: VariantControl=V_z1_w2_hti1
  hygrothermal model : carnotUIBK/wall_zone/hygrothermal model  VariantControl=V_z1_w2_m2  t0=z.t_ini  reflectground=0.2  abs_emiss=[const.absorption_2 const.emission_2 const.emission_1]  xmesh=const.parameter.xmesh_hygro  X=const.parameter.X  d=const.parameter.d  lambda=const.parameter.lambda_hygro  rho=const.parameter.rho_hygro  cp=const.parameter.cp_hygro  mu=const.parameter.mu  ufs=const.parameter.ufs  FSF_u=const.parameter.FSF_u  FSF_phi=const.parameter.FSF_phi  FSF_dudphi=const.parameter.FSF_dudphi  FSF_k=const.parameter.FSF_k  K_kleff=const.parameter.K_kleff  K_u=const.parameter.K_u  K_kl=const.parameter.K_kl  FSF_length=const.parameter.FSF_length  K_length=const.parameter.K_length  T_ini=const.parameter.T_ini_hygro  Phi_ini=const.parameter.Phi_ini_hygro  T_source=const.parameter.T_source  Phi_source=const.parameter.Phi_source  Tdactive=const.parameter.T_dactive  Phidactive=const.parameter.Phi_dactive
      link override alpha_e/alpha_e_AMBIENT: VariantControl=V_z1_w2_hte0
      link override alpha_e/alpha_e_GROUND: VariantControl=V_z1_w2_hte1
      link override alpha_e/alpha_e_INTERNAL: VariantControl=V_z1_w2_hte2
      link override alpha_e/alpha_e_INTERNAL/alpha_i/alpha_i_down: VariantControl=V_z1_w2_hti2
      link override alpha_e/alpha_e_INTERNAL/alpha_i/alpha_i_horizontal: VariantControl=V_z1_w2_hti0
      link override alpha_e/alpha_e_INTERNAL/alpha_i/alpha_i_up: VariantControl=V_z1_w2_hti1
      link override alpha_e/alpha_e_NEIGHBOUR: VariantControl=V_z1_w2_hte3
      link override alpha_e/alpha_e_NEIGHBOUR/alpha_i/alpha_i_down: VariantControl=V_z1_w2_hti2
      link override alpha_e/alpha_e_NEIGHBOUR/alpha_i/alpha_i_horizontal: VariantControl=V_z1_w2_hti0
      link override alpha_e/alpha_e_NEIGHBOUR/alpha_i/alpha_i_up: VariantControl=V_z1_w2_hti1
      link override alpha_i/alpha_i_down: VariantControl=V_z1_w2_hti2
      link override alpha_i/alpha_i_horizontal: VariantControl=V_z1_w2_hti0
      link override alpha_i/alpha_i_up: VariantControl=V_z1_w2_hti1
  "[S]" : Outport  VectorParamsAs1DForOutWhenUnconnected=off
  theta_out : Outport  Port=2  VectorParamsAs1DForOutWhenUnconnected=off

== system building_PHPP_v4/BUILDING/ZONE_1/wall_3 ==
  WDB : Inport
  GDB : Inport  Port=2
  NDB : Inport  Port=3
  AIB : Inport  Port=4
  Qdot_in : Inport  Port=5
  Qdot_sol : Inport  Port=6
  EMPTY : carnotUIBK/wall_zone/EMPTY  VariantControl=(default)
  R-C model : carnotUIBK/wall_zone/R-C model  VariantControl=V_z1_w3_m1  t0=z.t_ini  d=fliplr(const.parameter.xmesh_beu)  cond=fliplr(const.parameter.lambda)  cwall=fliplr(const.parameter.cp)  rho=fliplr(const.parameter.rho)  reflectground=0.2  abs_emiss=[const.absorption_2 const.emission_2 const.emission_1]  tau=const.parameter.tau  dactive=const.parameter.d_active
      link override alpha_e/alpha_e_AMBIENT: VariantControl=V_z1_w3_hte0
      link override alpha_e/alpha_e_GROUND: VariantControl=V_z1_w3_hte1
      link override alpha_e/alpha_e_INTERNAL: VariantControl=V_z1_w3_hte2
      link override alpha_e/alpha_e_INTERNAL/alpha_i/alpha_i_down: VariantControl=V_z1_w3_hti2
      link override alpha_e/alpha_e_INTERNAL/alpha_i/alpha_i_horizontal: VariantControl=V_z1_w3_hti0
      link override alpha_e/alpha_e_INTERNAL/alpha_i/alpha_i_up: VariantControl=V_z1_w3_hti1
      link override alpha_e/alpha_e_NEIGHBOUR: VariantControl=V_z1_w3_hte3
      link override alpha_e/alpha_e_NEIGHBOUR/alpha_i/alpha_i_down: VariantControl=V_z1_w3_hti2
      link override alpha_e/alpha_e_NEIGHBOUR/alpha_i/alpha_i_horizontal: VariantControl=V_z1_w3_hti0
      link override alpha_e/alpha_e_NEIGHBOUR/alpha_i/alpha_i_up: VariantControl=V_z1_w3_hti1
      link override alpha_i/alpha_i_down: VariantControl=V_z1_w3_hti2
      link override alpha_i/alpha_i_horizontal: VariantControl=V_z1_w3_hti0
      link override alpha_i/alpha_i_up: VariantControl=V_z1_w3_hti1
  UA : carnotUIBK/wall_zone/UA  VariantControl=V_z1_w3_m0  U=const.parameter.U
      link override Rse/AMBIENT: VariantControl=V_z1_w3_hte0
      link override Rse/GROUND: VariantControl=V_z1_w3_hte1
      link override Rse/INTERNAL: VariantControl=V_z1_w3_hte2
      link override Rse/NEIGHBOUR: VariantControl=V_z1_w3_hte3
      link override Rsi/down: VariantControl=V_z1_w3_hti2
      link override Rsi/horizontal: VariantControl=V_z1_w3_hti0
      link override Rsi/up: VariantControl=V_z1_w3_hti1
  hygrothermal model : carnotUIBK/wall_zone/hygrothermal model  VariantControl=V_z1_w3_m2  t0=z.t_ini  reflectground=0.2  abs_emiss=[const.absorption_2 const.emission_2 const.emission_1]  xmesh=const.parameter.xmesh_hygro  X=const.parameter.X  d=const.parameter.d  lambda=const.parameter.lambda_hygro  rho=const.parameter.rho_hygro  cp=const.parameter.cp_hygro  mu=const.parameter.mu  ufs=const.parameter.ufs  FSF_u=const.parameter.FSF_u  FSF_phi=const.parameter.FSF_phi  FSF_dudphi=const.parameter.FSF_dudphi  FSF_k=const.parameter.FSF_k  K_kleff=const.parameter.K_kleff  K_u=const.parameter.K_u  K_kl=const.parameter.K_kl  FSF_length=const.parameter.FSF_length  K_length=const.parameter.K_length  T_ini=const.parameter.T_ini_hygro  Phi_ini=const.parameter.Phi_ini_hygro  T_source=const.parameter.T_source  Phi_source=const.parameter.Phi_source  Tdactive=const.parameter.T_dactive  Phidactive=const.parameter.Phi_dactive
      link override alpha_e/alpha_e_AMBIENT: VariantControl=V_z1_w3_hte0
      link override alpha_e/alpha_e_GROUND: VariantControl=V_z1_w3_hte1
      link override alpha_e/alpha_e_INTERNAL: VariantControl=V_z1_w3_hte2
      link override alpha_e/alpha_e_INTERNAL/alpha_i/alpha_i_down: VariantControl=V_z1_w3_hti2
      link override alpha_e/alpha_e_INTERNAL/alpha_i/alpha_i_horizontal: VariantControl=V_z1_w3_hti0
      link override alpha_e/alpha_e_INTERNAL/alpha_i/alpha_i_up: VariantControl=V_z1_w3_hti1
      link override alpha_e/alpha_e_NEIGHBOUR: VariantControl=V_z1_w3_hte3
      link override alpha_e/alpha_e_NEIGHBOUR/alpha_i/alpha_i_down: VariantControl=V_z1_w3_hti2
      link override alpha_e/alpha_e_NEIGHBOUR/alpha_i/alpha_i_horizontal: VariantControl=V_z1_w3_hti0
      link override alpha_e/alpha_e_NEIGHBOUR/alpha_i/alpha_i_up: VariantControl=V_z1_w3_hti1
      link override alpha_i/alpha_i_down: VariantControl=V_z1_w3_hti2
      link override alpha_i/alpha_i_horizontal: VariantControl=V_z1_w3_hti0
      link override alpha_i/alpha_i_up: VariantControl=V_z1_w3_hti1
  "[S]" : Outport  VectorParamsAs1DForOutWhenUnconnected=off
  theta_out : Outport  Port=2  VectorParamsAs1DForOutWhenUnconnected=off

== system building_PHPP_v4/BUILDING/ZONE_1/wall_4 ==
  WDB : Inport
  GDB : Inport  Port=2
  NDB : Inport  Port=3
  AIB : Inport  Port=4
  Qdot_in : Inport  Port=5
  Qdot_sol : Inport  Port=6
  EMPTY : carnotUIBK/wall_zone/EMPTY  VariantControl=(default)
  R-C model : carnotUIBK/wall_zone/R-C model  VariantControl=V_z1_w4_m1  t0=z.t_ini  d=fliplr(const.parameter.xmesh_beu)  cond=fliplr(const.parameter.lambda)  cwall=fliplr(const.parameter.cp)  rho=fliplr(const.parameter.rho)  reflectground=0.2  abs_emiss=[const.absorption_2 const.emission_2 const.emission_1]  tau=const.parameter.tau  dactive=const.parameter.d_active
      link override alpha_e/alpha_e_AMBIENT: VariantControl=V_z1_w4_hte0
      link override alpha_e/alpha_e_GROUND: VariantControl=V_z1_w4_hte1
      link override alpha_e/alpha_e_INTERNAL: VariantControl=V_z1_w4_hte2
      link override alpha_e/alpha_e_INTERNAL/alpha_i/alpha_i_down: VariantControl=V_z1_w4_hti2
      link override alpha_e/alpha_e_INTERNAL/alpha_i/alpha_i_horizontal: VariantControl=V_z1_w4_hti0
      link override alpha_e/alpha_e_INTERNAL/alpha_i/alpha_i_up: VariantControl=V_z1_w4_hti1
      link override alpha_e/alpha_e_NEIGHBOUR: VariantControl=V_z1_w4_hte3
      link override alpha_e/alpha_e_NEIGHBOUR/alpha_i/alpha_i_down: VariantControl=V_z1_w4_hti2
      link override alpha_e/alpha_e_NEIGHBOUR/alpha_i/alpha_i_horizontal: VariantControl=V_z1_w4_hti0
      link override alpha_e/alpha_e_NEIGHBOUR/alpha_i/alpha_i_up: VariantControl=V_z1_w4_hti1
      link override alpha_i/alpha_i_down: VariantControl=V_z1_w4_hti2
      link override alpha_i/alpha_i_horizontal: VariantControl=V_z1_w4_hti0
      link override alpha_i/alpha_i_up: VariantControl=V_z1_w4_hti1
  UA : carnotUIBK/wall_zone/UA  VariantControl=V_z1_w4_m0  U=const.parameter.U
      link override Rse/AMBIENT: VariantControl=V_z1_w4_hte0
      link override Rse/GROUND: VariantControl=V_z1_w4_hte1
      link override Rse/INTERNAL: VariantControl=V_z1_w4_hte2
      link override Rse/NEIGHBOUR: VariantControl=V_z1_w4_hte3
      link override Rsi/down: VariantControl=V_z1_w4_hti2
      link override Rsi/horizontal: VariantControl=V_z1_w4_hti0
      link override Rsi/up: VariantControl=V_z1_w4_hti1
  hygrothermal model : carnotUIBK/wall_zone/hygrothermal model  VariantControl=V_z1_w4_m2  t0=z.t_ini  reflectground=0.2  abs_emiss=[const.absorption_2 const.emission_2 const.emission_1]  xmesh=const.parameter.xmesh_hygro  X=const.parameter.X  d=const.parameter.d  lambda=const.parameter.lambda_hygro  rho=const.parameter.rho_hygro  cp=const.parameter.cp_hygro  mu=const.parameter.mu  ufs=const.parameter.ufs  FSF_u=const.parameter.FSF_u  FSF_phi=const.parameter.FSF_phi  FSF_dudphi=const.parameter.FSF_dudphi  FSF_k=const.parameter.FSF_k  K_kleff=const.parameter.K_kleff  K_u=const.parameter.K_u  K_kl=const.parameter.K_kl  FSF_length=const.parameter.FSF_length  K_length=const.parameter.K_length  T_ini=const.parameter.T_ini_hygro  Phi_ini=const.parameter.Phi_ini_hygro  T_source=const.parameter.T_source  Phi_source=const.parameter.Phi_source  Tdactive=const.parameter.T_dactive  Phidactive=const.parameter.Phi_dactive
      link override alpha_e/alpha_e_AMBIENT: VariantControl=V_z1_w4_hte0
      link override alpha_e/alpha_e_GROUND: VariantControl=V_z1_w4_hte1
      link override alpha_e/alpha_e_INTERNAL: VariantControl=V_z1_w4_hte2
      link override alpha_e/alpha_e_INTERNAL/alpha_i/alpha_i_down: VariantControl=V_z1_w4_hti2
      link override alpha_e/alpha_e_INTERNAL/alpha_i/alpha_i_horizontal: VariantControl=V_z1_w4_hti0
      link override alpha_e/alpha_e_INTERNAL/alpha_i/alpha_i_up: VariantControl=V_z1_w4_hti1
      link override alpha_e/alpha_e_NEIGHBOUR: VariantControl=V_z1_w4_hte3
      link override alpha_e/alpha_e_NEIGHBOUR/alpha_i/alpha_i_down: VariantControl=V_z1_w4_hti2
      link override alpha_e/alpha_e_NEIGHBOUR/alpha_i/alpha_i_horizontal: VariantControl=V_z1_w4_hti0
      link override alpha_e/alpha_e_NEIGHBOUR/alpha_i/alpha_i_up: VariantControl=V_z1_w4_hti1
      link override alpha_i/alpha_i_down: VariantControl=V_z1_w4_hti2
      link override alpha_i/alpha_i_horizontal: VariantControl=V_z1_w4_hti0
      link override alpha_i/alpha_i_up: VariantControl=V_z1_w4_hti1
  "[S]" : Outport  VectorParamsAs1DForOutWhenUnconnected=off
  theta_out : Outport  Port=2  VectorParamsAs1DForOutWhenUnconnected=off

== system building_PHPP_v4/BUILDING/ZONE_1/wall_5 ==
  WDB : Inport
  GDB : Inport  Port=2
  NDB : Inport  Port=3
  AIB : Inport  Port=4
  Qdot_in : Inport  Port=5
  Qdot_sol : Inport  Port=6
  EMPTY : carnotUIBK/wall_zone/EMPTY  VariantControl=(default)
  R-C model : carnotUIBK/wall_zone/R-C model  VariantControl=V_z1_w5_m1  t0=z.t_ini  d=fliplr(const.parameter.xmesh_beu)  cond=fliplr(const.parameter.lambda)  cwall=fliplr(const.parameter.cp)  rho=fliplr(const.parameter.rho)  reflectground=0.2  abs_emiss=[const.absorption_2 const.emission_2 const.emission_1]  tau=const.parameter.tau  dactive=const.parameter.d_active
      link override alpha_e/alpha_e_AMBIENT: VariantControl=V_z1_w5_hte0
      link override alpha_e/alpha_e_GROUND: VariantControl=V_z1_w5_hte1
      link override alpha_e/alpha_e_INTERNAL: VariantControl=V_z1_w5_hte2
      link override alpha_e/alpha_e_INTERNAL/alpha_i/alpha_i_down: VariantControl=V_z1_w5_hti2
      link override alpha_e/alpha_e_INTERNAL/alpha_i/alpha_i_horizontal: VariantControl=V_z1_w5_hti0
      link override alpha_e/alpha_e_INTERNAL/alpha_i/alpha_i_up: VariantControl=V_z1_w5_hti1
      link override alpha_e/alpha_e_NEIGHBOUR: VariantControl=V_z1_w5_hte3
      link override alpha_e/alpha_e_NEIGHBOUR/alpha_i/alpha_i_down: VariantControl=V_z1_w5_hti2
      link override alpha_e/alpha_e_NEIGHBOUR/alpha_i/alpha_i_horizontal: VariantControl=V_z1_w5_hti0
      link override alpha_e/alpha_e_NEIGHBOUR/alpha_i/alpha_i_up: VariantControl=V_z1_w5_hti1
      link override alpha_i/alpha_i_down: VariantControl=V_z1_w5_hti2
      link override alpha_i/alpha_i_horizontal: VariantControl=V_z1_w5_hti0
      link override alpha_i/alpha_i_up: VariantControl=V_z1_w5_hti1
  UA : carnotUIBK/wall_zone/UA  VariantControl=V_z1_w5_m0  U=const.parameter.U
      link override Rse/AMBIENT: VariantControl=V_z1_w5_hte0
      link override Rse/GROUND: VariantControl=V_z1_w5_hte1
      link override Rse/INTERNAL: VariantControl=V_z1_w5_hte2
      link override Rse/NEIGHBOUR: VariantControl=V_z1_w5_hte3
      link override Rsi/down: VariantControl=V_z1_w5_hti2
      link override Rsi/horizontal: VariantControl=V_z1_w5_hti0
      link override Rsi/up: VariantControl=V_z1_w5_hti1
  hygrothermal model : carnotUIBK/wall_zone/hygrothermal model  VariantControl=V_z1_w5_m2  t0=z.t_ini  reflectground=0.2  abs_emiss=[const.absorption_2 const.emission_2 const.emission_1]  xmesh=const.parameter.xmesh_hygro  X=const.parameter.X  d=const.parameter.d  lambda=const.parameter.lambda_hygro  rho=const.parameter.rho_hygro  cp=const.parameter.cp_hygro  mu=const.parameter.mu  ufs=const.parameter.ufs  FSF_u=const.parameter.FSF_u  FSF_phi=const.parameter.FSF_phi  FSF_dudphi=const.parameter.FSF_dudphi  FSF_k=const.parameter.FSF_k  K_kleff=const.parameter.K_kleff  K_u=const.parameter.K_u  K_kl=const.parameter.K_kl  FSF_length=const.parameter.FSF_length  K_length=const.parameter.K_length  T_ini=const.parameter.T_ini_hygro  Phi_ini=const.parameter.Phi_ini_hygro  T_source=const.parameter.T_source  Phi_source=const.parameter.Phi_source  Tdactive=const.parameter.T_dactive  Phidactive=const.parameter.Phi_dactive
      link override alpha_e/alpha_e_AMBIENT: VariantControl=V_z1_w5_hte0
      link override alpha_e/alpha_e_GROUND: VariantControl=V_z1_w5_hte1
      link override alpha_e/alpha_e_INTERNAL: VariantControl=V_z1_w5_hte2
      link override alpha_e/alpha_e_INTERNAL/alpha_i/alpha_i_down: VariantControl=V_z1_w5_hti2
      link override alpha_e/alpha_e_INTERNAL/alpha_i/alpha_i_horizontal: VariantControl=V_z1_w5_hti0
      link override alpha_e/alpha_e_INTERNAL/alpha_i/alpha_i_up: VariantControl=V_z1_w5_hti1
      link override alpha_e/alpha_e_NEIGHBOUR: VariantControl=V_z1_w5_hte3
      link override alpha_e/alpha_e_NEIGHBOUR/alpha_i/alpha_i_down: VariantControl=V_z1_w5_hti2
      link override alpha_e/alpha_e_NEIGHBOUR/alpha_i/alpha_i_horizontal: VariantControl=V_z1_w5_hti0
      link override alpha_e/alpha_e_NEIGHBOUR/alpha_i/alpha_i_up: VariantControl=V_z1_w5_hti1
      link override alpha_i/alpha_i_down: VariantControl=V_z1_w5_hti2
      link override alpha_i/alpha_i_horizontal: VariantControl=V_z1_w5_hti0
      link override alpha_i/alpha_i_up: VariantControl=V_z1_w5_hti1
  "[S]" : Outport  VectorParamsAs1DForOutWhenUnconnected=off
  theta_out : Outport  Port=2  VectorParamsAs1DForOutWhenUnconnected=off
